simulink model "baseband_tb"  (R2021b)
settings: Solver=FixedStepDiscrete  StartTime=0.0  StopTime=10.0  RelTol=1e-3
model workspace (MATLAB code in the model file):
  | cmdLim = Simulink.Parameter;
  | cmdLim.Value = 15;
  | cmdLim.Description = 'Limit for controlling the maximum surface command angle.';
  | cmdLim.Min = 0;
  | cmdLim.Max = 90;
  | cmdLim.DocUnits = 'deg';
  | 
  | dispGain = Simulink.Parameter;
  | dispGain.Value = 0.75;
  | dispGain.Description = 'Gain applied to the displacement error.';
  | dispGain.Min = 0;
  | dispGain.Max = [];
  | dispGain.DocUnits = 'deg/sec/deg';
  | 
  | dispLim = Simulink.Parameter;
  | dispLim.Value = 30;
  | dispLim.Description = 'Limit for controlling the maximum commanded angle.';
  | dispLim.Min = 0;
  | dispLim.Max = 180;
  | dispLim.DocUnits = 'deg';
  | 
  | intGain = Simulink.Parameter;
  | intGain.Value = 0.5;
  | intGain.Description = 'Gain applied to the integral error.';
  | intGain.Min = 0;
  | intGain.Max = [];
  | intGain.DocUnits = 'deg/sec/deg/sec';
  | 
  | intLim = Simulink.Parameter;
  | intLim.Value = 5;
  | intLim.Description = 'Limit for controlling the maximum commanded angle.';
  | intLim.Min = 0;
  | intLim.Max = 90;
  | intLim.DocUnits = 'deg';
  | 
  | rateGain = Simulink.Parameter;
  | rateGain.Value = 2;
  | rateGain.Description = 'Gain applied to the rate error.';
  | rateGain.Min = 0;
  | rateGain.Max = [];
  | rateGain.DocUnits = 'deg/deg/sec';
  | 
  | rateLim = Simulink.Parameter;
  | rateLim.Value = 6;
  | rateLim.Description = 'Limit for controlling the maximum commanded angle.';
  | rateLim.Min = 0;
  | rateLim.Max = 180;
  | rateLim.DocUnits = 'deg/sec';
  | 
  | hdgGain = Simulink.Parameter;
  | hdgGain.Value = 0.015;
values from neighbouring files (symbols this model uses):
  bb_ini = baseband_init()    [run_baseband_tb.m]    (also in run_v2x_baseband_tb.m = v2x_baseband_init(); run_v2x_modem_tb.m = v2x_baseband_init())
  seed = 123    [run_baseband_tb.m]    (also in run_v2x_baseband_tb.m; run_v2x_data_tb.m; run_v2x_modem_tb.m)
  Ts = 1    [run_baseband_tb.m]    (also in run_v2x_baseband_tb.m; run_v2x_data_tb.m = ini.T; run_v2x_modem_tb.m = ini.T)
undefined symbols (not defined in the file or in its folder): rsgenpoly
libraries: commsink2 x5, commrandsrc3 x2, commblkcod2 x2, commdigbbndpm3 x2, commsequence2 x2, commsync2 x1
settings Model: RequirementInfo={} %GIDa_fe9045fd_0412_4b6e_8206_617cc20e6fde  FPTRunName=Active  Creator=jacob  LastModifiedBy=jacob
settings SolverCC: AlgebraicLoopSolver=TrustRegion  AutoInsertRateTranBlk=on
settings DataIOCC: SaveOutput=off  SignalLogging=off  DSMLogging=off  SaveTime=off
settings OptimizationCC: DefaultParameterBehavior=Inlined  UseDivisionForNetSlopeComputation=on  GainParamInheritBuiltInType=on  UseFloatMulNetSlope=on  UseSpecifiedMinMax=on  InlineInvariantSignals=on  EnhancedBackFolding=on  PassReuseOutputArgsAs=Individual arguments  ZeroExternalMemoryAtStartup=off  ZeroInternalMemoryAtStartup=off  NoFixptDivByZeroProtection=on  EfficientFloat2IntCast=on  LifeSpan=1  OptimizeBlockOrder=speed  DifferentSizesBufferReuse=on  OptimizationCustomize=off  EfficientTunableParamExpr=on
settings DebuggingCC: SFUnexpectedBacktrackingDiag=warning  SFNoUnconditionalDefaultTransitionDiag=warning  SFExecutionAtInitializationDiag=none  ArithmeticOperatorsInVariantConditions=warning
settings HardwareCC: ProdLongLongMode=on
settings SFSimCC: MATLABDynamicMemAlloc=off
settings RTWCC: Description=Embedded Coder  SystemTargetFile=ert.tlc  TemplateMakefile=ert_default_tmf  BuildConfiguration=Faster Runs
settings CodeAppCC: ForceParamTrailComments=on  IgnoreCustomStorageClasses=off  OperatorAnnotations=on  SimulinkDataObjDesc=on  SFDataObjDesc=on  CustomSymbolStrGlobalVar=rt$N$M  CustomSymbolStrType=$N$M  CustomSymbolStrFcn=$N$M$F  CustomSymbolStrMacro=$N$M  InsertBlockDesc=on  EnableCustomComments=on  ReqsInCode=on
settings ERTTargetCC: TargetLangStandard=C99 (ISO)  UtilityFuncGeneration=Shared location  MultiwordLength=2048  GenerateSampleERTMain=on  IncludeMdlTerminateFcn=off  CombineSignalStateStructs=on  SuppressErrorStatus=on  SupportAbsoluteTime=off  SupportNonFinite=off  SupportComplex=off  InlinedParameterPlacement=NonHierarchical  ERTCustomFileTemplate=example_file_process.tlc  ERTFilePackagingFormat=CompactWithDataFile
settings ConfigComp: CovScope=ReferencedModels  CovSaveName=covdata_rollAP  CovMetricSettings=dcmtrwe  CovHTMLOptions=-sRT=1 -aTS=1 -bRG=1 -bTC=1 -hTR=1 -nFC=0 -scm=1 -bcm=1 -xEv=0  CovSaveCumulativeToWorkspaceVar=on  CovSaveSingleToWorkspaceVar=on  CovCumulativeVarName=covCumulativeData_rollAP  CovReportOnPause=off  CovExternalEMLEnable=off  CovSFcnEnable=off

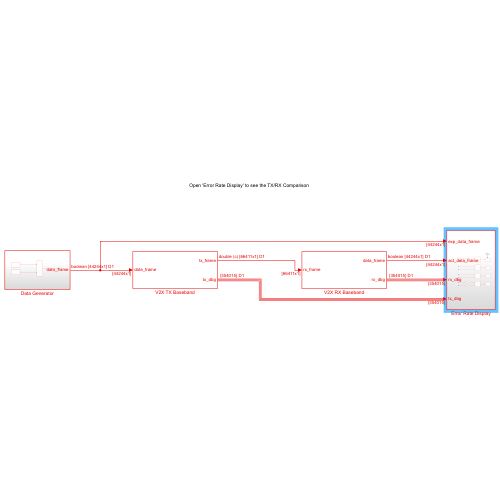
[thumbnail: Simulink's stored preview of the top-level diagram]
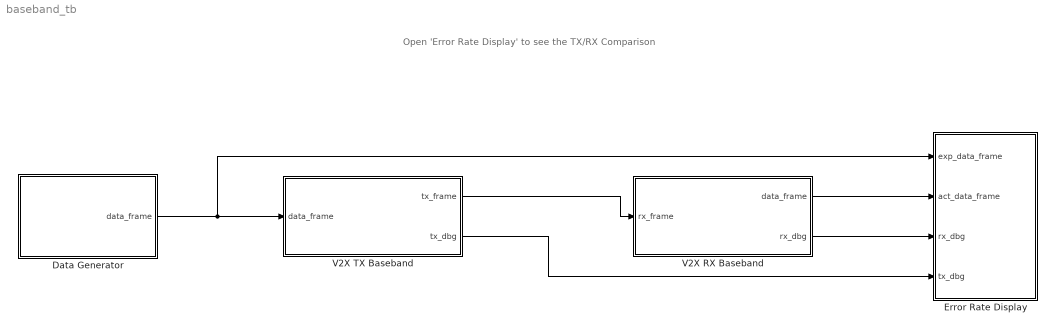
== system baseband_tb ==
  note: Open 'Error Rate Display' to see the TX/RX Comparison
  Data Generator : Subsystem
  Error Rate Display : Subsystem
  V2X RX Baseband : Subsystem
      mask init:
      | ini = baseband_init();
  V2X TX Baseband : Subsystem
      mask init:
      | ini = baseband_init();
  wires:
  Data Generator/1(data_frame) -> Error Rate Display/1(exp_data_frame), V2X TX Baseband/1(data_frame)
  V2X TX Baseband/1(tx_frame) -> V2X RX Baseband/1(rx_frame)
  V2X RX Baseband/1(data_frame) -> Error Rate Display/2(act_data_frame)
  V2X RX Baseband/2(rx_dbg) -> Error Rate Display/3(rx_dbg)
  V2X TX Baseband/2(tx_dbg) -> Error Rate Display/4(tx_dbg)

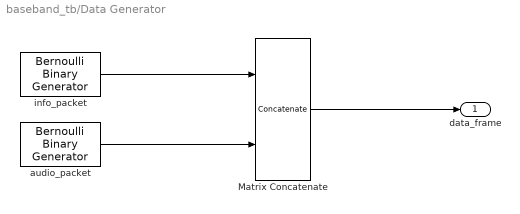
== system baseband_tb/Data Generator ==
  Matrix Concatenate : Concatenate  Mode=Multidimensional array
  audio_packet : commrandsrc3/Bernoulli Binary Generator  ProbabilityOfZero=0.5  SeedSource=Parameter  Seed=seed  SampleTime=Ts/bb_ini.audio_len  SamplesPerFrame=bb_ini.audio_len  OutputDataType=boolean  SimulateUsing=Interpreted execution
  info_packet : commrandsrc3/Bernoulli Binary Generator  ProbabilityOfZero=0.5  SeedSource=Parameter  Seed=seed  SampleTime=Ts/bb_ini.info_len  SamplesPerFrame=bb_ini.info_len  OutputDataType=boolean  SimulateUsing=Interpreted execution
  data_frame : Outport
  wires:
  info_packet/1 -> Matrix Concatenate/1
  audio_packet/1 -> Matrix Concatenate/2
  Matrix Concatenate/1 -> data_frame/1

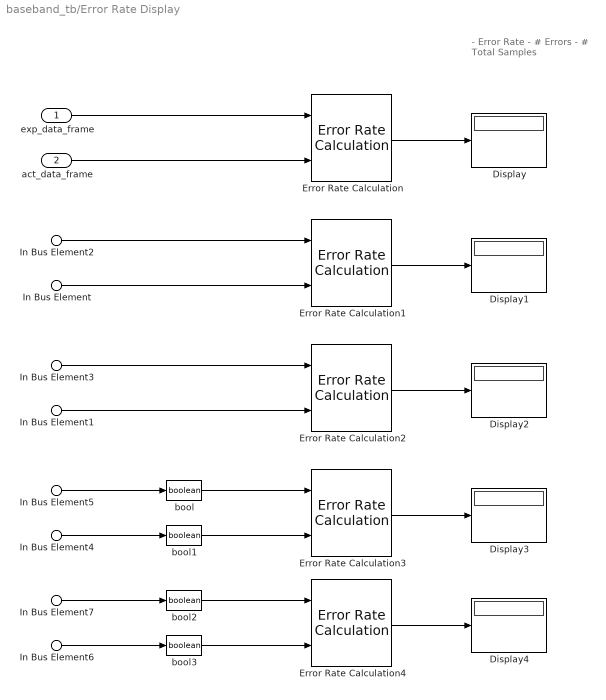
== system baseband_tb/Error Rate Display ==
  note: - Error Rate
      | - # Errors
      | - # Total Samples
  exp_data_frame : Inport
  act_data_frame : Inport  Port=2
  In Bus Element : Inport  Port=3  PortName=rx_dbg  Element=rx_in
  In Bus Element1 : Inport  Port=3  PortName=rx_dbg  Element=demapper_in
  In Bus Element4 : Inport  Port=3  PortName=rx_dbg  Element=decoder_in
  In Bus Element6 : Inport  Port=3  PortName=rx_dbg  Element=descrambler_in
  In Bus Element2 : Inport  Port=4  PortName=tx_dbg  Element=tx_out
  In Bus Element3 : Inport  Port=4  PortName=tx_dbg  Element=mapper_out
  In Bus Element5 : Inport  Port=4  PortName=tx_dbg  Element=encoder_out
  In Bus Element7 : Inport  Port=4  PortName=tx_dbg  Element=scrambler_out
  Display{,1..4} (5 alike) : Display
  Error Rate Calculation{,1..4} (5 alike) : commsink2/Error Rate Calculation  N=0  st_delay=0  cp_mode=Entire frame  subframe=[]  PMode=Port  WsName=ErrorVec  RsMode2=off  stop=off  numErr=100  maxBits=1e6
  bool{,1..3} (4 alike) : DataTypeConversion  OutDataTypeStr=boolean
  wires:
  Error Rate Calculation/1 -> Display/1
  exp_data_frame/1 -> Error Rate Calculation/1
  act_data_frame/1 -> Error Rate Calculation/2
  Error Rate Calculation1/1 -> Display1/1
  In Bus Element2/1 -> Error Rate Calculation1/1
  In Bus Element/1 -> Error Rate Calculation1/2
  In Bus Element1/1 -> Error Rate Calculation2/2
  In Bus Element3/1 -> Error Rate Calculation2/1
  Error Rate Calculation2/1 -> Display2/1
  Error Rate Calculation3/1 -> Display3/1
  bool/1 -> Error Rate Calculation3/1
  In Bus Element5/1 -> bool/1
  In Bus Element4/1 -> bool1/1
  bool1/1 -> Error Rate Calculation3/2
  Error Rate Calculation4/1 -> Display4/1
  In Bus Element7/1 -> bool2/1
  bool3/1 -> Error Rate Calculation4/2
  bool2/1 -> Error Rate Calculation4/1
  In Bus Element6/1 -> bool3/1

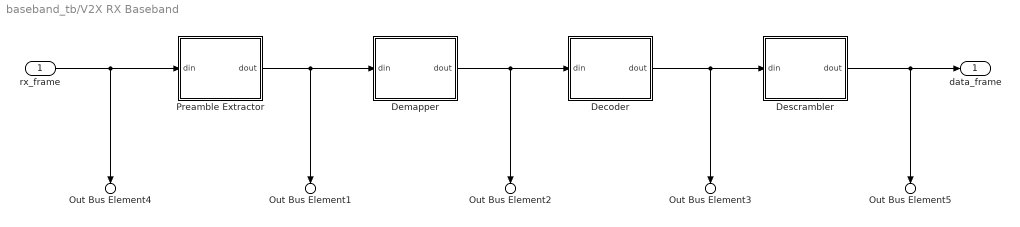
== system baseband_tb/V2X RX Baseband ==
  rx_frame : Inport
  Decoder : Subsystem
  Demapper : Subsystem
  Descrambler : Subsystem
  Preamble Extractor : Subsystem
  data_frame : Outport
  Out Bus Element4 : Outport  Port=2  PortName=rx_dbg  Element=rx_in
  Out Bus Element1 : Outport  Port=2  PortName=rx_dbg  Element=demapper_in
  Out Bus Element2 : Outport  Port=2  PortName=rx_dbg  Element=decoder_in
  Out Bus Element3 : Outport  Port=2  PortName=rx_dbg  Element=descrambler_in
  Out Bus Element5 : Outport  Port=2  PortName=rx_dbg  Element=rx_out
  wires:
  rx_frame/1 -> Preamble Extractor/1(din), Out Bus Element4/1
  Preamble Extractor/1(dout) -> Out Bus Element1/1, Demapper/1(din)
  Demapper/1(dout) -> Decoder/1(din), Out Bus Element2/1
  Decoder/1(dout) -> Out Bus Element3/1, Descrambler/1(din)
  Descrambler/1(dout) -> Out Bus Element5/1, data_frame/1

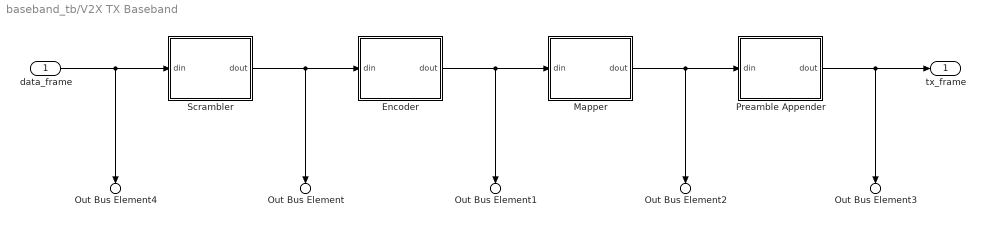
== system baseband_tb/V2X TX Baseband ==
  data_frame : Inport
  Encoder : Subsystem
  Mapper : Subsystem
  Preamble Appender : Subsystem
  Scrambler : Subsystem
  tx_frame : Outport
  Out Bus Element4 : Outport  Port=2  PortName=tx_dbg  Element=tx_in
  Out Bus Element : Outport  Port=2  PortName=tx_dbg  Element=scrambler_out
  Out Bus Element1 : Outport  Port=2  PortName=tx_dbg  Element=encoder_out
  Out Bus Element2 : Outport  Port=2  PortName=tx_dbg  Element=mapper_out
  Out Bus Element3 : Outport  Port=2  PortName=tx_dbg  Element=tx_out
  wires:
  data_frame/1 -> Out Bus Element4/1, Scrambler/1(din)
  Scrambler/1(dout) -> Out Bus Element/1, Encoder/1(din)
  Encoder/1(dout) -> Mapper/1(din), Out Bus Element1/1
  Mapper/1(dout) -> Preamble Appender/1(din), Out Bus Element2/1
  Preamble Appender/1(dout) -> Out Bus Element3/1, tx_frame/1

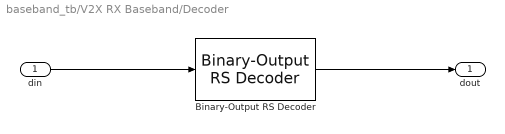
== system baseband_tb/V2X RX Baseband/Decoder ==
  din : Inport
  Binary-Output RS Decoder : commblkcod2/Binary-Output RS Decoder  n=ini.encoder_n  k=ini.encoder_k  specShortening=off  shortenedK=3  specGenPoly=off  genPoly=rsgenpoly(7, 3, [], [], 'double')  specPrimPoly=off  prPoly='X^3 + X + 1'  specPuncture=off  punctVec=[ones(2,1); zeros(2,1)]  specErasurePort=off  showNumErr=off  outDType=Same as input
      settings: SourceProductBaseCode=CM
  dout : Outport
  wires:
  Binary-Output RS Decoder/1 -> dout/1
  din/1 -> Binary-Output RS Decoder/1

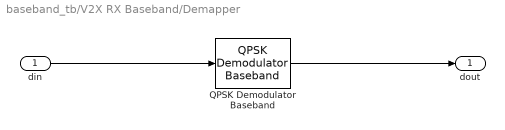
== system baseband_tb/V2X RX Baseband/Demapper ==
  din : Inport
  QPSK Demodulator Baseband : commdigbbndpm3/QPSK Demodulator Baseband  OutType=Bit  DecType=Hard decision  VarSource=Dialog  Variance=1  Dec=Gray  Ph=pi/4  outDtype1=Inherit via internal rule  outDtype2=Inherit via internal rule  derotateFactorWordLen=16  derotateFactorDataTypeStr=Inherit: Same word length as input  derotateFactorLastDataTypeStr=Inherit: Same word length as input
  dout : Outport
  wires:
  QPSK Demodulator Baseband/1 -> dout/1
  din/1 -> QPSK Demodulator Baseband/1

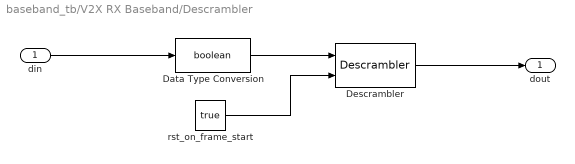
== system baseband_tb/V2X RX Baseband/Descrambler ==
  din : Inport
  Data Type Conversion : DataTypeConversion  OutDataTypeStr=boolean
  Descrambler : commsequence2/Descrambler  M=2  poly=ini.scramb_tap  iniStaSource=Dialog Parameter  ini_sta=ini.scramb_seed  resetViaPort=on
      settings: SourceProductBaseCode=CM
  rst_on_frame_start : Constant  Value=true  SampleTime=-1
  dout : Outport
  wires:
  rst_on_frame_start/1 -> Descrambler/2
  Descrambler/1 -> dout/1
  din/1 -> Data Type Conversion/1
  Data Type Conversion/1 -> Descrambler/1

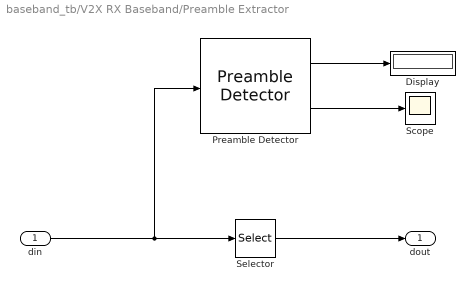
== system baseband_tb/V2X RX Baseband/Preamble Extractor ==
  din : Inport
  Display : Display
  Preamble Detector : commsync2/Preamble Detector  Input=Symbol  Preamble=ini.preamble  Threshold=ini.detect_thresh  DetectionMetricOutput=on  Detections=First  SimulateUsing=Interpreted execution
      settings: SourceProductBaseCode=CM
  Scope : Scope
  Selector : Selector  InputPortWidth=ini.rx_frame_len  IndexOptions=Starting index (dialog)  Indices=ini.preamble_len + 1  OutputSizes=ini.demapper_out_len
  dout : Outport
  wires:
  din/1 -> Selector/1, Preamble Detector/1
  Preamble Detector/1 -> Display/1
  Preamble Detector/2 -> Scope/1
  Selector/1 -> dout/1

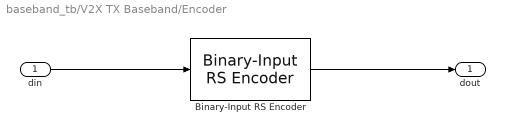
== system baseband_tb/V2X TX Baseband/Encoder ==
  din : Inport
  Binary-Input RS Encoder : commblkcod2/Binary-Input RS Encoder  n=ini.encoder_n  k=ini.encoder_k  specShortening=off  shortenedK=3  specGenPoly=off  genPoly=rsgenpoly(7, 3, [], [], 'double')  specPrimPoly=off  prPoly='X^3 + X + 1'  specPuncture=off  punctVec=[ones(2,1); zeros(2,1)]  outDType=Same as input
      settings: SourceProductBaseCode=CM
  dout : Outport
  wires:
  din/1 -> Binary-Input RS Encoder/1
  Binary-Input RS Encoder/1 -> dout/1

== system baseband_tb/V2X TX Baseband/Mapper ==
  din : Inport
  QPSK Modulator Baseband : commdigbbndpm3/QPSK Modulator Baseband  InType=Bit  Enc=Gray  Ph=pi/4  outDtype=double  outWordLen=16  outUDDataType=sfix(16)  outFracLenMode=Best precision  outFracLen=15  outDataTypeStr=double  outLastDataTypeStr=double
  dout : Outport
  wires:
  QPSK Modulator Baseband/1 -> dout/1
  din/1 -> QPSK Modulator Baseband/1

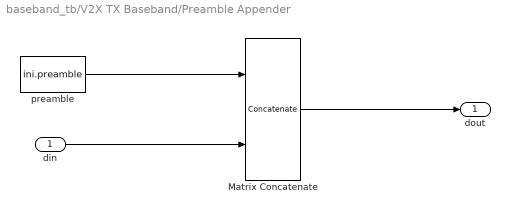
== system baseband_tb/V2X TX Baseband/Preamble Appender ==
  din : Inport
  Matrix Concatenate : Concatenate  Mode=Multidimensional array
  preamble : Constant  Value=ini.preamble  VectorParams1D=off  SampleTime=-1
  dout : Outport
  wires:
  preamble/1 -> Matrix Concatenate/1
  din/1 -> Matrix Concatenate/2
  Matrix Concatenate/1 -> dout/1

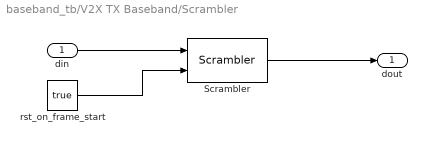
== system baseband_tb/V2X TX Baseband/Scrambler ==
  din : Inport
  Scrambler : commsequence2/Scrambler  M=2  poly=ini.scramb_tap  iniStaSource=Dialog Parameter  ini_sta=ini.scramb_seed  resetViaPort=on
      settings: SourceProductBaseCode=CM
  rst_on_frame_start : Constant  Value=true  SampleTime=-1
  dout : Outport
  wires:
  rst_on_frame_start/1 -> Scrambler/2
  Scrambler/1 -> dout/1
  din/1 -> Scrambler/1
